simulink model "taskx_multivariablesystem"  (R2017b)
settings: Solver=VariableStepAuto  StartTime=0.0  StopTime=100  RelTol=1e-3
values from neighbouring files (symbols this model uses):
  alpha = [alpha1; alpha2]    [OAC_LA_Ass2.m]
  beta = [beta1; beta2]    [OAC_LA_Ass2.m]
  gamma = [gamma1; gamma2]    [OAC_LA_Ass2.m]
  h = evalin('base','h')    [MPC_function.m]    (also in OAC_LA_Ass2.m = [h01; h02])
  k = [k1; k2]    [OAC_LA_Ass2.m]
  Ts = 0.5    [OAC_LA_Ass2.m]
undefined symbols (not defined in the file or in its folder): F, Fx, G, Gx
settings Model: Creator=lukastotschnig  LastModifiedBy=lukastotschnig

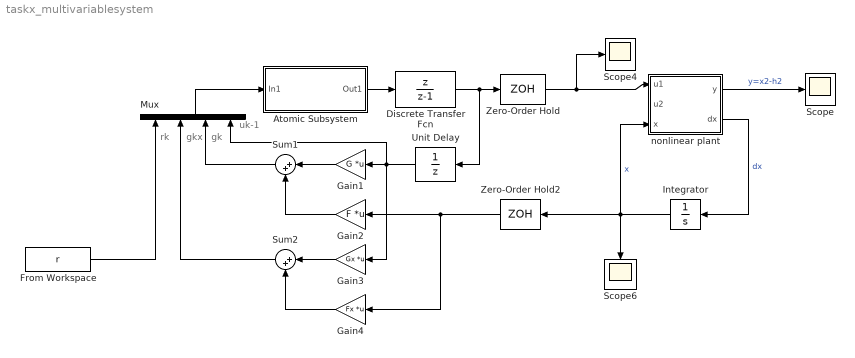
== system taskx_multivariablesystem ==
  note: uk-1
  note: gk
  note: gkx
  note: rk
  Atomic Subsystem : Subsystem  TreatAsAtomicUnit=on  SystemSampleTime=Ts
  Discrete Transfer Fcn : DiscreteTransferFcn  Numerator=[1 0]  Denominator=[1 -1]  SampleTime=Ts
  From Workspace : FromWorkspace  VariableName=r  SampleTime=Ts
  Gain1 : Gain  Gain=G  Multiplication=Matrix(K*u)
  Gain2 : Gain  Gain=F  Multiplication=Matrix(K*u)
  Gain3 : Gain  Gain=Gx  Multiplication=Matrix(K*u)
  Gain4 : Gain  Gain=Fx  Multiplication=Matrix(K*u)
  Integrator : Integrator  InitialCondition=h
  Mux : Mux
  Scope : Scope
  Scope4 : Scope
  Scope6 : Scope
  Sum1 : Sum  Inputs=|++
  Sum2 : Sum  Inputs=|++
  Unit Delay : UnitDelay  SampleTime=Ts
  Zero-Order Hold : ZeroOrderHold  SampleTime=Ts
  Zero-Order Hold2 : ZeroOrderHold  SampleTime=Ts
  nonlinear plant : MATLAB Function  TreatAsAtomicUnit=on
  wires:
  nonlinear plant/2(dx) -> Integrator/1  "dx"
  Integrator/1 -> Zero-Order Hold2/1, Scope6/1, nonlinear plant/3(x)  "x"
  Discrete Transfer Fcn/1 -> Unit Delay/1, Zero-Order Hold/1
  Unit Delay/1 -> Gain3/1, Mux/4, Gain1/1
  Gain1/1 -> Sum1/1
  Gain2/1 -> Sum1/2
  Zero-Order Hold2/1 -> Gain4/1, Gain2/1
  Zero-Order Hold/1 -> Scope4/1, nonlinear plant/1(u1)
  nonlinear plant/1(y) -> Scope/1  "y=x2-h2"
  Mux/1 -> Atomic Subsystem/1(In1)
  Atomic Subsystem/1(Out1) -> Discrete Transfer Fcn/1
  Gain4/1 -> Sum2/2
  Gain3/1 -> Sum2/1
  Sum1/1 -> Mux/3
  Sum2/1 -> Mux/2
  From Workspace/1 -> Mux/1

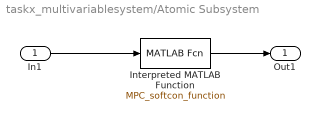
== system taskx_multivariablesystem/Atomic Subsystem ==
  In1 : Inport
  Interpreted MATLAB Function : MATLABFcn  MATLABFcn=MPC_softcon_function
  Out1 : Outport
  wires:
  In1/1 -> Interpreted MATLAB Function/1
  Interpreted MATLAB Function/1 -> Out1/1

== matlab function taskx_multivariablesystem/nonlinear plant ==
  data: y output; dx output; u1 input; u2 input; x input; k parameter; alpha parameter; beta parameter; gamma parameter; h parameter
function [y, dx]= fcn(u1,u2,x,k,alpha, beta, gamma,h)
    
    % calculate input quantity
    if (beta(1)+gamma(1)*u1) <= 0
        zp1 = 0;
        disp('zp1 = 0');
    else
        zp1 = alpha(1) + sqrt( beta(1)+gamma(1)*u1 );
    end
    
    if (beta(2)+gamma(2)*u2) <= 0
        zp2 = 0;
        disp('zp2 = 0');
    else
        zp2 = alpha(2) + sqrt( beta(2)+gamma(2)*u2 );
    end
    
    % nonlinear plant description
   dx1 = -k(1)*sqrt(x(1)) + zp1;
   dx2 = -k(2)*sqrt(x(2)) + k(1)*sqrt(x(1))+zp2;
   
   dx = [dx1; dx2];
   y = x(2)-h(2);

end
